simulink model "Controller_Design_Using_Pole_Positioning"  (R2023a)
settings: Solver=VariableStepAuto  StartTime=0.0  StopTime=10.0  RelTol=1e-3
undefined symbols (not defined in the file): A1, B1, k
settings Model: Creator=demo  LastModifiedBy=demo

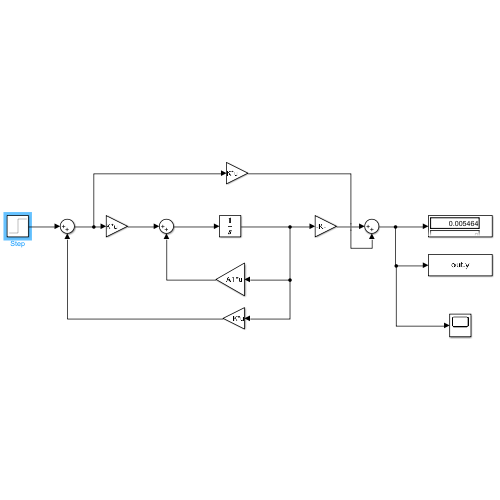
[thumbnail: Simulink's stored preview of the top-level diagram]
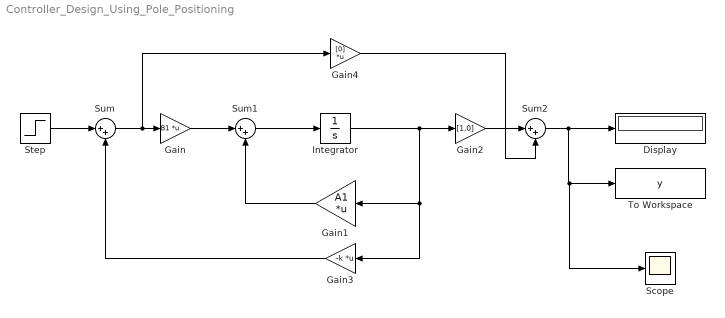
== system Controller_Design_Using_Pole_Positioning ==
  Display : Display
  Gain : Gain  Gain=B1  Multiplication=Matrix(K*u)
  Gain1 : Gain  Gain=A1  Multiplication=Matrix(K*u)
  Gain2 : Gain  Gain=[1,0]
  Gain3 : Gain  Gain=-k  Multiplication=Matrix(K*u)
  Gain4 : Gain  Gain=[0]  Multiplication=Matrix(K*u)
  Integrator : Integrator
  Scope : Scope
  Step : Step  Time=0  SampleTime=0
  Sum : Sum  Inputs=|++
  Sum1 : Sum  Inputs=|++
  Sum2 : Sum  Inputs=|++
  To Workspace : ToWorkspace  VariableName=y  SampleTime=-1
  wires:
  Gain4/1 -> Sum2/2
  Gain2/1 -> Sum2/1
  Integrator/1 -> Gain3/1, Gain1/1, Gain2/1
  Gain/1 -> Sum1/1
  Gain1/1 -> Sum1/2
  Sum/1 -> Gain4/1, Gain/1
  Gain3/1 -> Sum/2
  Sum2/1 -> Display/1, Scope/1, To Workspace/1
  Step/1 -> Sum/1
  Sum1/1 -> Integrator/1
